simulink model "multiple_clock_tb"  (Simulink 7.1)
settings: Solver=ode45  StartTime=0.0  StopTime=200  RelTol=1e-3
undefined symbols (not defined in the file): d, dly
libraries: xbsIndex_r4 x92, xbsReplacements_r4 x8, xbsCopyrightNotice_r4 x1
(part 2 of 2)

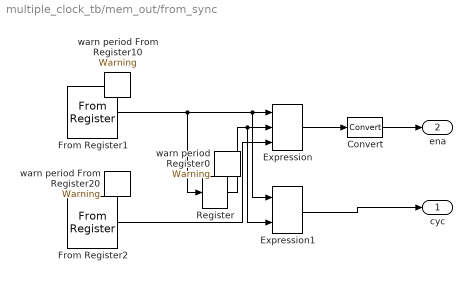
== system multiple_clock_tb/mem_out/from_sync ==
  Convert : xbsIndex_r4/Convert  arith_type=Boolean  n_bits=8  bin_pt=6  quantization=Truncate  overflow=Wrap  en=off  latency=0  dbl_ovrd=off  pipeline=off  block_type=convert
      settings: xl_area=[0, 0, 0, 0, 0, 0, 0]  block_version=VER_STRING_GOES_HERE
  Expression : xbsIndex_r4/Expression  expression=(d^dly)&ena  align_bp=on  en=off  latency=0  precision=User Defined  arith_type=Unsigned  n_bits=1  bin_pt=0  dbl_ovrd=off  block_type=expr
      settings: xl_area=[0, 0, 0, 0, 0, 0, 0]  block_version=VER_STRING_GOES_HERE
  Expression1 : xbsIndex_r4/Expression  expression=d^dly  align_bp=on  en=off  latency=0  precision=User Defined  arith_type=Unsigned  n_bits=1  bin_pt=0  dbl_ovrd=off  block_type=expr
      settings: xl_area=[0, 0, 0, 0, 0, 0, 0]  block_version=VER_STRING_GOES_HERE
  From Register1 : xbsIndex_r4/From Register  shared_memory_name='mem_clk'  init=0  period=period  ownership=Owned and initialized elsewhere  arith_type=Unsigned  n_bits=1  bin_pt=0  dbl_ovrd=off  block_type=fromreg
      settings: AttributesFormatString=<< %<shared_memory_name> >>  infoedit="Register block that reads data to a shared memory register.  Delay of one sample period."  xl_area=[0, 0, 0, 0, 0, 0, 0]  block_version=VER_STRING_GOES_HERE
  From Register2 : xbsIndex_r4/From Register  shared_memory_name='mem_ena'  init=0  period=period  ownership=Owned and initialized elsewhere  arith_type=Unsigned  n_bits=1  bin_pt=0  dbl_ovrd=off  block_type=fromreg
      settings: AttributesFormatString=<< %<shared_memory_name> >>  infoedit="Register block that reads data to a shared memory register.  Delay of one sample period."  xl_area=[0, 0, 0, 0, 0, 0, 0]  block_version=VER_STRING_GOES_HERE
  Register : xbsIndex_r4/Register  init=1  rst=off  en=off  dbl_ovrd=off  block_type=register
      settings: xl_area=[0, 0, 0, 0, 0, 0, 0]  block_version=VER_STRING_GOES_HERE
  warn period From Register10 : xbsReplacements_r4/Warning  SystemSampleTime=-1  period=period
  warn period From Register20 : xbsReplacements_r4/Warning  SystemSampleTime=-1  period=period
  warn period Register0 : xbsReplacements_r4/Warning  SystemSampleTime=-1  period=period
  cyc : Outport  OutDataType=sfix(16)  OutScaling=2^0
  ena : Outport  Port=2  OutDataType=sfix(16)  OutScaling=2^0
  wires:
  From Register1/1 -> Register/1, Expression/1, Expression1/1
  Register/1 -> Expression/2, Expression1/2
  From Register2/1 -> Expression/3
  Expression/1 -> Convert/1
  Convert/1 -> ena/1
  Expression1/1 -> cyc/1

== system multiple_clock_tb/reg_in/To Sync ==
  note: toggle flop
  ena : Inport  OutDataType=sfix(16)  OutScaling=2^0
  Assert : xbsIndex_r4/Assert  Orientation=left  assert_type=off  type_source=Explicitly  arith_type="Signed  (2's comp)"  n_bits=16  bin_pt=14  assert_rate=on  rate_source=Explicitly  period=period  output_port=on  block_type=assert
      settings: infoedit=Asserts a user-defined sample rate and/or type on a signal.<P><P>Hardware notes: In hardware this block costs nothing.  block_version=VER_STRING_GOES_HERE
  Constant1 : xbsIndex_r4/Constant  arith_type=Boolean  const=1  n_bits=1  bin_pt=0  explicit_period=off  period=1  equ=P=C  opselect=C  inp2=PCIN>>17  opr=+  inp1=P  carry=CIN  dbl_ovrd=off  block_type=constant
      settings: block_version=VER_STRING_GOES_HERE
  Expression : xbsIndex_r4/Expression  expression=~i  align_bp=on  en=off  latency=0  precision=User Defined  arith_type=Unsigned  n_bits=1  bin_pt=0  dbl_ovrd=off  block_type=expr
      settings: xl_area=[0, 0, 0, 0, 0, 0, 0]  block_version=VER_STRING_GOES_HERE
  Register : xbsIndex_r4/Register  init=0  rst=off  en=off  dbl_ovrd=off  block_type=register
      settings: xl_area=[0, 0, 0, 0, 0, 0, 0]  block_version=VER_STRING_GOES_HERE
  To Register1 : xbsIndex_r4/To Register  shared_memory_name='reg_clk'  init=0  ownership=Locally owned and initialized  explicit_data_type=off  arith_type=Unsigned  n_bits=0  bin_pt=0  dbl_ovrd=off  block_type=toreg
      settings: AttributesFormatString=<< %<shared_memory_name> >>  infoedit="Register block that writes data to a shared memory register.  Delay of one sample period."  xl_area=[0, 0, 0, 0, 0, 0, 0]  block_version=VER_STRING_GOES_HERE
  To Register2 : xbsIndex_r4/To Register  shared_memory_name='reg_ena'  init=0  ownership=Locally owned and initialized  explicit_data_type=off  arith_type=Unsigned  n_bits=0  bin_pt=0  dbl_ovrd=off  block_type=toreg
      settings: AttributesFormatString=<< %<shared_memory_name> >>  infoedit="Register block that writes data to a shared memory register.  Delay of one sample period."  xl_area=[0, 0, 0, 0, 0, 0, 0]  block_version=VER_STRING_GOES_HERE
  warn period Register0 : xbsReplacements_r4/Warning  SystemSampleTime=-1  period=period
  cyc : Outport  OutDataType=sfix(16)  OutScaling=2^0
  eo : Outport  Port=2  OutDataType=sfix(16)  OutScaling=2^0
  wires:
  Expression/1 -> Register/1
  Constant1/1 -> To Register1/2, To Register2/2
  Register/1 -> To Register1/1, Assert/1
  ena/1 -> To Register2/1
  To Register1/1 -> cyc/1
  To Register2/1 -> eo/1
  Assert/1 -> Expression/1

== system multiple_clock_tb/reg_out/From Sync ==
  Expression : xbsIndex_r4/Expression  expression=(d^dly)&ena  align_bp=on  en=off  latency=0  precision=User Defined  arith_type=Unsigned  n_bits=1  bin_pt=0  dbl_ovrd=off  block_type=expr
      settings: xl_area=[0, 0, 0, 0, 0, 0, 0]  block_version=VER_STRING_GOES_HERE
  From Register1 : xbsIndex_r4/From Register  shared_memory_name='reg_clk'  init=0  period=period  ownership=Owned and initialized elsewhere  arith_type=Unsigned  n_bits=1  bin_pt=0  dbl_ovrd=off  block_type=fromreg
      settings: AttributesFormatString=<< %<shared_memory_name> >>  infoedit="Register block that reads data to a shared memory register.  Delay of one sample period."  xl_area=[0, 0, 0, 0, 0, 0, 0]  block_version=VER_STRING_GOES_HERE
  From Register2 : xbsIndex_r4/From Register  shared_memory_name='reg_ena'  init=0  period=period  ownership=Owned and initialized elsewhere  arith_type=Unsigned  n_bits=1  bin_pt=0  dbl_ovrd=off  block_type=fromreg
      settings: AttributesFormatString=<< %<shared_memory_name> >>  infoedit="Register block that reads data to a shared memory register.  Delay of one sample period."  xl_area=[0, 0, 0, 0, 0, 0, 0]  block_version=VER_STRING_GOES_HERE
  Register : xbsIndex_r4/Register  init=1  rst=off  en=off  dbl_ovrd=off  block_type=register
      settings: xl_area=[0, 0, 0, 0, 0, 0, 0]  block_version=VER_STRING_GOES_HERE
  warn period From Register10 : xbsReplacements_r4/Warning  SystemSampleTime=-1  period=period
  warn period From Register20 : xbsReplacements_r4/Warning  SystemSampleTime=-1  period=period
  warn period Register0 : xbsReplacements_r4/Warning  SystemSampleTime=-1  period=period
  ena : Outport  OutDataType=sfix(16)  OutScaling=2^0
  cyc : Outport  Port=2  OutDataType=sfix(16)  OutScaling=2^0
  wires:
  From Register1/1 -> Expression/1, Register/1, cyc/1
  Register/1 -> Expression/2
  From Register2/1 -> Expression/3
  Expression/1 -> ena/1

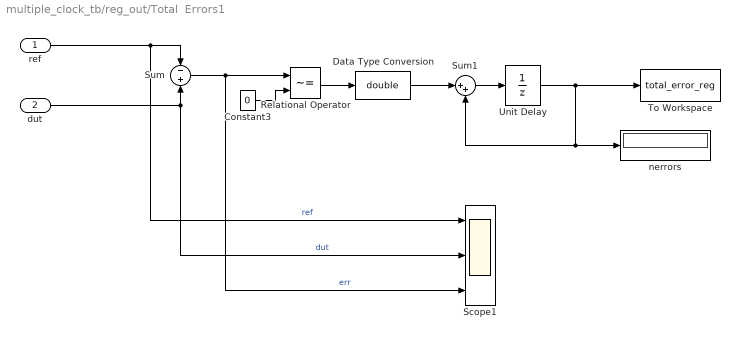
== system multiple_clock_tb/reg_out/Total  Errors1 ==
  ref : Inport  OutDataType=sfix(16)  OutScaling=2^0
  dut : Inport  Port=2  OutDataType=sfix(16)  OutScaling=2^0
  Constant3 : Constant  Value=0  OutDataType=sfix(16)  OutScaling=2^0
  Data Type Conversion : DataTypeConversion  OutDataTypeMode=double  OutDataType=sfix(16)  OutScaling=2^0  OutDataTypeStr=double  SaturateOnIntegerOverflow=on  RndMeth=Zero
  Relational Operator : RelationalOperator  Operator=~=  LogicOutDataTypeMode=Specify via dialog  LogicDataType=sint(32)  OutDataTypeStr=sint(32)
  Scope1 : Scope  NumInputPorts=3
      settings: YMin=-5~-5~-5  YMax=5~5~5
  Sum : Sum  Inputs=-|+  OutDataType=sfix(16)  OutScaling=2^0  SaturateOnIntegerOverflow=on
  Sum1 : Sum  Inputs=|++  OutDataType=sfix(16)  OutScaling=2^0  SaturateOnIntegerOverflow=on
  To Workspace : ToWorkspace  VariableName=total_error_reg  SampleTime=-1  SaveFormat=Array
      settings: MaxDataPoints=1
  Unit Delay : UnitDelay
  nerrors : Display
  wires:
  Sum1/1 -> Unit Delay/1
  ref/1 -> Sum/1, Scope1/1  "ref"
  Sum/1 -> Scope1/3, Relational Operator/1  "err"
  dut/1 -> Sum/2, Scope1/2  "dut"
  Relational Operator/1 -> Data Type Conversion/1
  Constant3/1 -> Relational Operator/2
  Data Type Conversion/1 -> Sum1/1
  Unit Delay/1 -> To Workspace/1, nerrors/1, Sum1/2
